simulink model "pi1semanti"  (R2020a)
settings: Solver=VariableStepAuto  StartTime=0.0  StopTime=1  RelTol=1e-3
values from neighbouring files (symbols this model uses):
  B = 0.003032    [motorfase_valores.m]
  flux = 0.12    [motorfase_valores.m]
  inddiff = 0.0125    [motorfase_valores.m]
  J = 0.0042    [motorfase_valores.m]
  p = 3    [motorfase_valores.m]
  R = 2.3    [motorfase_valores.m]
libraries: powerlib x13, eePwmGenerator x1, simulink x1
settings Model: Creator=ryt14  LastModifiedBy=ryt14
settings SolverCC: ZeroCrossAlgorithm=Adaptive
settings DebuggingCC: IgnoredZcDiagnostic=none

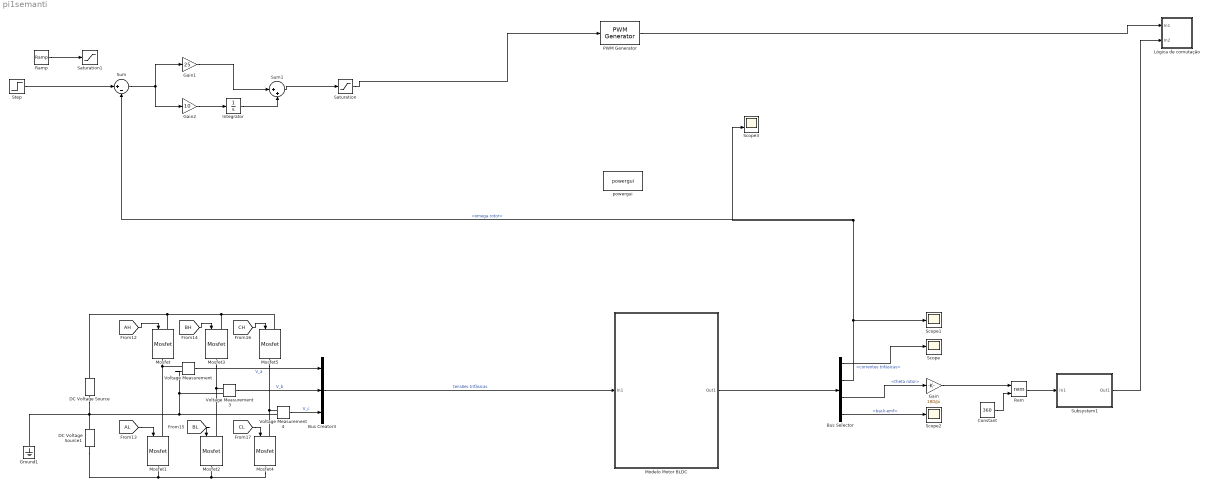
== system pi1semanti ==
  Bus Creator3 : BusCreator  Inputs=3
  Bus Selector : BusSelector  OutputSignals=correntes trifásicas,omega rotor,theta rotor,back-emf
  Constant : Constant  Value=360
  DC Voltage Source : powerlib/Electrical Sources/DC Voltage Source  Amplitude=75  Measurements=None
  DC Voltage Source1 : powerlib/Electrical Sources/DC Voltage Source  Amplitude=75  Measurements=None
  Gain : Gain  Gain=180/pi
  Gain1 : Gain  Gain=25
  Gain2 : Gain  Gain=10
  Ground1 : powerlib/Elements/Ground  LConnTagsString=a
  Integrator : Integrator
  Lógica de comutação : Subsystem
  Modelo Motor BLDC : Subsystem
  Mosfet{,1..5} (6 alike) : powerlib/Power Electronics/Mosfet  Ron=0.1  Lon=0  Rd=0.01  Vfd=0  IC=0  Rs=1e5  Cs=inf  Measurements=off
  PWM Generator : eePwmGenerator/PWM Generator  CarrCount=Up  Tper=0.001  Ts=5e-5
  Ramp : simulink/Sources/Ramp  slope=10  start=0  InitialOutput=0
  Rem : Math  Operator=rem  SaturateOnIntegerOverflow=on
  Saturation : Saturate  UpperLimit=1  LowerLimit=0
  Saturation1 : Saturate  UpperLimit=50  LowerLimit=0
  Scope : Scope
  Scope1 : Scope
  Scope2 : Scope
  Scope3 : Scope  NumInputPorts=2
  Step : Step  Time=0  After=100  SampleTime=0
  Subsystem1 : Subsystem
  Sum : Sum  Inputs=|+-
  Sum1 : Sum  Inputs=|++
  Voltage Measurement : powerlib/Measurements/Voltage Measurement  PhasorSimulation=off  OutputType=Complex  PSBequivalent=0
  Voltage Measurement3 : powerlib/Measurements/Voltage Measurement  PhasorSimulation=off  OutputType=Complex  PSBequivalent=0
  Voltage Measurement4 : powerlib/Measurements/Voltage Measurement  PhasorSimulation=off  OutputType=Complex  PSBequivalent=0
  powergui : powerlib/powergui  Priority=1  SimulationMode=Continuous  SampleTime=50e-6  frequency=60  Iterations=50  frequencyindice=0  Pbase=100e6  ErrMax=1e-4  UnitsV=kV  UnitsW=MW  buscounter=0  FunctionMessages=off  echomessages=off  EnableUseOfTLC=off  CurrentSourceSwitches=off  DisableSnubberDevices=off  DisableRonSwitches=off  DisableVfSwitches=off  DisplayEquations=off  AutomaticDiscreteSolvers=off  SolverType=Tustin/Backward Euler (TBE)  Interpol=off  ExternalGateDelay=off  methode=off  Ts=100  x0status=blocks  SPID=on  SwTol=0  HookPort=off  NonlinearTolerance=1e-4  nMaxIteration=100  ContinueOnMaxIteration=off  RestoreLinks=warning  ResistiveCurrentMeasurement=off  Frange=[0:2:500]  Ylog=off  Xlog=on  ShowGrid=off  save=off  variable=ZData  structure=0  ZoomFFT=off  StartTime=0.0  cycles=1  DisplayStyle=1  fundamental=60  FreqAxis=off  MaxFrequency=1000  frequencyindicesteady=1  RmsSteady=1  display=off
  wires:
  Voltage Measurement3/1 -> Bus Creator3/2  "V_b"
  Voltage Measurement4/1 -> Bus Creator3/3  "V_c"
  Voltage Measurement/1 -> Bus Creator3/1  "V_a"
  Bus Creator3/1 -> Modelo Motor BLDC/1(In1)  "tensões trifásicas"
  Modelo Motor BLDC/1(Out1) -> Bus Selector/1
  Gain/1 -> Rem/1
  Bus Selector/3 -> Gain/1  "<theta rotor>"
  Constant/1 -> Rem/2
  Rem/1 -> Subsystem1/1(In1)
  Bus Selector/2 -> Scope3/2, Sum/2, Scope1/1  "<omega rotor>"
  [AH] -> Mosfet/1
  [BH] -> Mosfet3/1
  [CH] -> Mosfet5/1
  [BL] -> Mosfet2/1
  [CL] -> Mosfet4/1
  [AL] -> Mosfet1/1
  Bus Selector/1 -> Scope/1  "<correntes trifásicas>"
  Bus Selector/4 -> Scope2/1  "<back-emf>"
  Sum/1 -> Gain1/1, Gain2/1
  PWM Generator/1 -> Lógica de comutação/1(In1)
  Subsystem1/1(Out1) -> Lógica de comutação/2(In2)
  Sum1/1 -> Saturation/1
  Saturation/1 -> PWM Generator/1
  Gain1/1 -> Sum1/1
  Integrator/1 -> Sum1/2
  Gain2/1 -> Integrator/1
  Ramp/1 -> Saturation1/1
  Step/1 -> Sum/1
  connections:
  Mosfet/RConn1 -- Mosfet1/LConn1 -- Voltage Measurement/LConn1
  Mosfet3/RConn1 -- Mosfet2/LConn1 -- Voltage Measurement3/LConn1
  Mosfet5/RConn1 -- Mosfet4/LConn1 -- Voltage Measurement4/LConn1
  Mosfet/LConn1 -- Mosfet5/LConn1 -- Mosfet3/LConn1 -- DC Voltage Source/RConn1
  DC Voltage Source/LConn1 -- Ground1/LConn1 -- DC Voltage Source1/RConn1 -- Voltage Measurement3/LConn2 -- Voltage Measurement/LConn2 -- Voltage Measurement4/LConn2
  Mosfet4/RConn1 -- DC Voltage Source1/LConn1 -- Mosfet1/RConn1 -- Mosfet2/RConn1

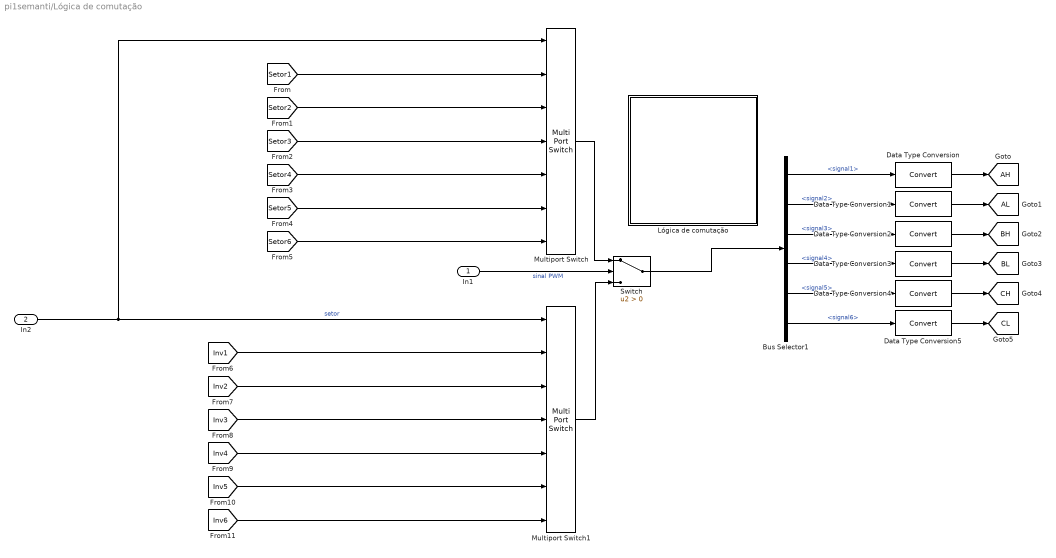
== system pi1semanti/Lógica de comutação ==
  In1 : Inport
  In2 : Inport  Port=2
  Bus Selector1 : BusSelector  OutputSignals=signal1,signal2,signal3,signal4,signal5,signal6
  Data Type Conversion{,1..5} (6 alike) : DataTypeConversion
  Lógica de comutação : Subsystem
  Multiport Switch : MultiPortSwitch  Inputs=6
  Multiport Switch1 : MultiPortSwitch  Inputs=6
  Switch : Switch  Criteria=u2 > Threshold
  tag scope: AH=global, AL=global, BH=global, BL=global, CH=global, CL=global
  wires:
  [Setor5] -> Multiport Switch/6
  [Inv4] -> Multiport Switch1/5
  [Setor1] -> Multiport Switch/2
  Data Type Conversion1/1 -> [AL]
  [Setor3] -> Multiport Switch/4
  Bus Selector1/2 -> Data Type Conversion1/1  "<signal2>"
  Data Type Conversion4/1 -> [CH]
  Switch/1 -> Bus Selector1/1
  [Setor6] -> Multiport Switch/7
  Bus Selector1/5 -> Data Type Conversion4/1  "<signal5>"
  Data Type Conversion/1 -> [AH]
  [Inv3] -> Multiport Switch1/4
  Data Type Conversion5/1 -> [CL]
  Bus Selector1/6 -> Data Type Conversion5/1  "<signal6>"
  Bus Selector1/1 -> Data Type Conversion/1  "<signal1>"
  [Inv2] -> Multiport Switch1/3
  Bus Selector1/3 -> Data Type Conversion2/1  "<signal3>"
  [Setor2] -> Multiport Switch/3
  [Inv1] -> Multiport Switch1/2
  Data Type Conversion3/1 -> [BL]
  Data Type Conversion2/1 -> [BH]
  In2/1 -> Multiport Switch1/1, Multiport Switch/1  "setor"
  Multiport Switch/1 -> Switch/1
  [Setor4] -> Multiport Switch/5
  [Inv6] -> Multiport Switch1/7
  [Inv5] -> Multiport Switch1/6
  Multiport Switch1/1 -> Switch/3
  Bus Selector1/4 -> Data Type Conversion3/1  "<signal4>"
  In1/1 -> Switch/2  "sinal PWM"

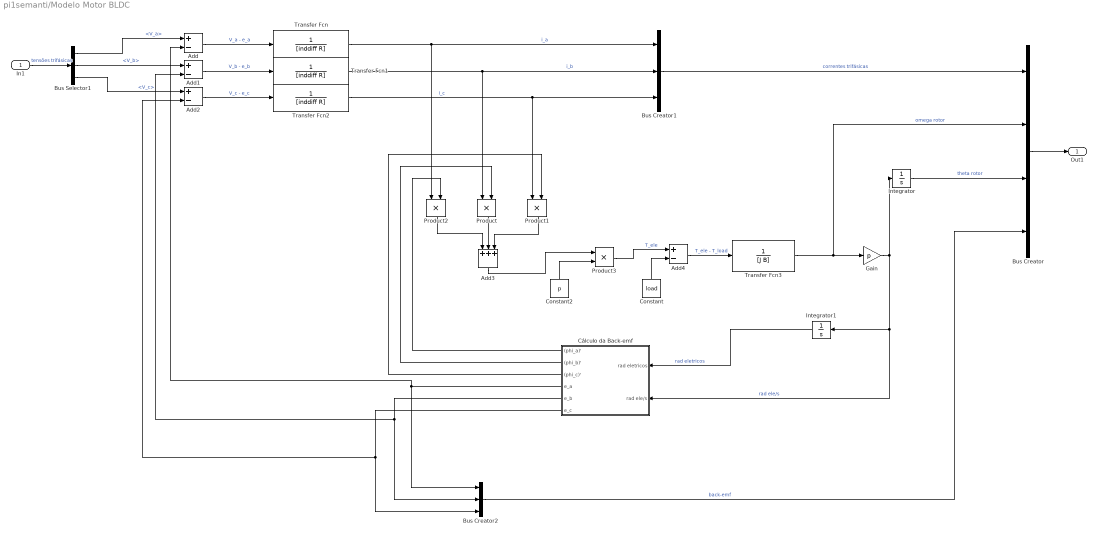
== system pi1semanti/Modelo Motor BLDC ==
  In1 : Inport
  Add{,1..2,4} (4 alike) : Sum  Inputs=+-
  Add3 : Sum  Inputs=+++
  Bus Creator : BusCreator  Inputs=4
  Bus Creator1 : BusCreator  Inputs=3
  Bus Creator2 : BusCreator  Inputs=3
  Bus Selector1 : BusSelector  OutputSignals=V_a,V_b,V_c
  Constant : Constant  Value=load
  Constant2 : Constant  Value=p
  Cálculo da Back-emf : Subsystem
  Gain : Gain  Gain=p
  Integrator : Integrator
  Integrator1 : Integrator
  Product : Product
  Product1 : Product
  Product2 : Product
  Product3 : Product  Inputs=**
  Transfer Fcn : TransferFcn  Denominator=[inddiff R]
  Transfer Fcn1 : TransferFcn  Denominator=[inddiff R]
  Transfer Fcn2 : TransferFcn  Denominator=[inddiff R]
  Transfer Fcn3 : TransferFcn  Denominator=[J B]
  Out1 : Outport
  wires:
  Add/1 -> Transfer Fcn/1  "V_a - e_a"
  Add2/1 -> Transfer Fcn2/1  "V_c - e_c"
  Constant/1 -> Add4/2
  Bus Selector1/2 -> Add1/1  "<V_b>"
  Bus Creator1/1 -> Bus Creator/1  "correntes trifásicas"
  Add1/1 -> Transfer Fcn1/1  "V_b - e_b"
  Product1/1 -> Add3/3
  Transfer Fcn1/1 -> Product/1, Bus Creator1/2  "i_b"
  Product2/1 -> Add3/1
  Product3/1 -> Add4/1  "T_ele"
  Bus Selector1/1 -> Add/1  "<V_a>"
  Transfer Fcn2/1 -> Product1/1, Bus Creator1/3  "i_c"
  Add4/1 -> Transfer Fcn3/1  "T_ele - T_load"
  Transfer Fcn/1 -> Product2/1, Bus Creator1/1  "i_a"
  Bus Selector1/3 -> Add2/1  "<V_c>"
  Bus Creator2/1 -> Bus Creator/4  "back-emf"
  Product/1 -> Add3/2
  In1/1 -> Bus Selector1/1  "tensões trifásicas"
  Gain/1 -> Integrator/1, Integrator1/1, Cálculo da Back-emf/2(rad ele/s)  "rad ele/s"
  Integrator/1 -> Bus Creator/3  "theta rotor"
  Bus Creator/1 -> Out1/1
  Add3/1 -> Product3/1
  Constant2/1 -> Product3/2
  Transfer Fcn3/1 -> Bus Creator/2, Gain/1  "omega rotor"
  Cálculo da Back-emf/6(e_c) -> Add2/2, Bus Creator2/3
  Cálculo da Back-emf/5(e_b) -> Add1/2, Bus Creator2/2
  Cálculo da Back-emf/4(e_a) -> Add/2, Bus Creator2/1
  Integrator1/1 -> Cálculo da Back-emf/1(rad eletricos)  "rad eletricos"
  Cálculo da Back-emf/1((phi_a)') -> Product2/2
  Cálculo da Back-emf/2((phi_b)') -> Product/2
  Cálculo da Back-emf/3((phi_c)') -> Product1/2

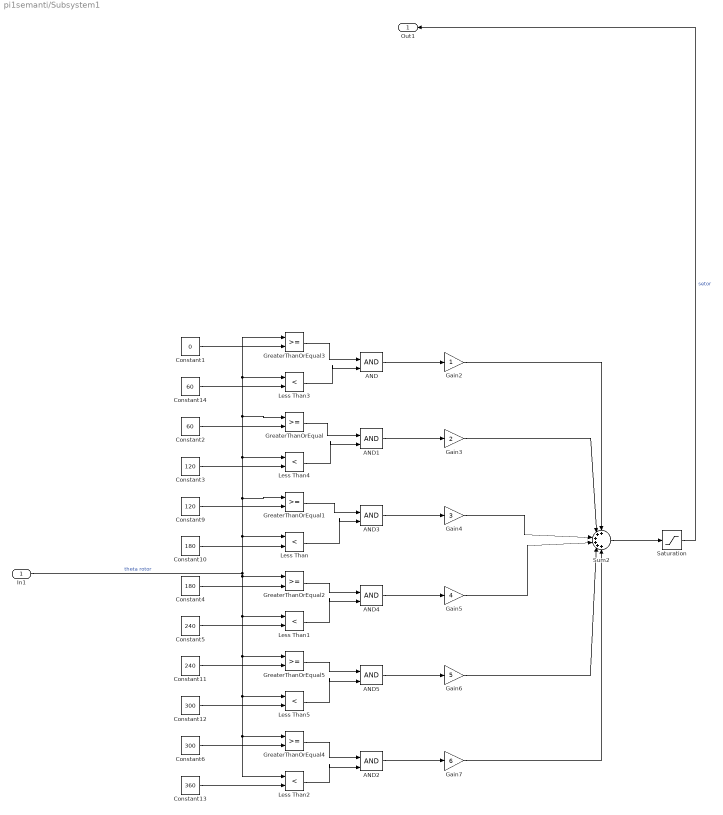
== system pi1semanti/Subsystem1 ==
  In1 : Inport
  AND{,1..5} (6 alike) : Logic  IconShape=distinctive  AllPortsSameDT=off  OutDataTypeStr=boolean
  Constant1 : Constant  Value=0
  Constant10 : Constant  Value=180
  Constant11 : Constant  Value=240
  Constant12 : Constant  Value=300
  Constant13 : Constant  Value=360
  Constant14 : Constant  Value=60
  Constant2 : Constant  Value=60
  Constant3 : Constant  Value=120
  Constant4 : Constant  Value=180
  Constant5 : Constant  Value=240
  Constant6 : Constant  Value=300
  Constant9 : Constant  Value=120
  Gain2 : Gain
  Gain3 : Gain  Gain=2
  Gain4 : Gain  Gain=3
  Gain5 : Gain  Gain=4
  Gain6 : Gain  Gain=5
  Gain7 : Gain  Gain=6
  GreaterThanOrEqual{,1..5} (6 alike) : RelationalOperator  OutDataTypeStr=boolean  RndMeth=Simplest
  Less Than{,1..5} (6 alike) : RelationalOperator  Operator=<  OutDataTypeStr=boolean  RndMeth=Simplest
  Saturation : Saturate  UpperLimit=6  LowerLimit=1
  Sum2 : Sum  Inputs=++++++
  Out1 : Outport
  wires:
  In1/1 -> Less Than/1, GreaterThanOrEqual1/1, GreaterThanOrEqual/1, GreaterThanOrEqual3/1, Less Than3/1, Less Than4/1, Less Than2/1, GreaterThanOrEqual4/1, Less Than5/1, GreaterThanOrEqual5/1, Less Than1/1, GreaterThanOrEqual2/1  "theta rotor"
  Less Than1/1 -> AND4/2
  Gain2/1 -> Sum2/1
  Sum2/1 -> Saturation/1
  Constant1/1 -> GreaterThanOrEqual3/2
  Constant9/1 -> GreaterThanOrEqual1/2
  Gain4/1 -> Sum2/3
  Gain5/1 -> Sum2/4
  AND/1 -> Gain2/1
  Constant13/1 -> Less Than2/2
  Constant2/1 -> GreaterThanOrEqual/2
  AND4/1 -> Gain5/1
  AND1/1 -> Gain3/1
  Less Than5/1 -> AND5/2
  Less Than/1 -> AND3/2
  GreaterThanOrEqual1/1 -> AND3/1
  Constant4/1 -> GreaterThanOrEqual2/2
  Gain3/1 -> Sum2/2
  Less Than2/1 -> AND2/2
  GreaterThanOrEqual5/1 -> AND5/1
  GreaterThanOrEqual/1 -> AND1/1
  Gain6/1 -> Sum2/5
  AND2/1 -> Gain7/1
  AND5/1 -> Gain6/1
  Less Than3/1 -> AND/2
  Constant11/1 -> GreaterThanOrEqual5/2
  Constant12/1 -> Less Than5/2
  Constant3/1 -> Less Than4/2
  Constant5/1 -> Less Than1/2
  Saturation/1 -> Out1/1  "setor"
  AND3/1 -> Gain4/1
  Constant14/1 -> Less Than3/2
  GreaterThanOrEqual2/1 -> AND4/1
  Less Than4/1 -> AND1/2
  Constant6/1 -> GreaterThanOrEqual4/2
  Constant10/1 -> Less Than/2
  GreaterThanOrEqual4/1 -> AND2/1
  Gain7/1 -> Sum2/6
  GreaterThanOrEqual3/1 -> AND/1

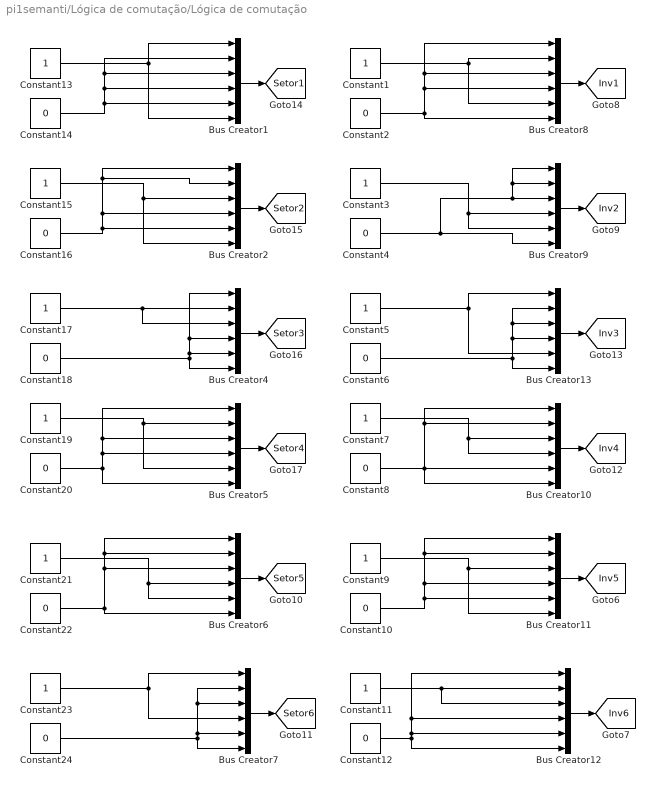
== system pi1semanti/Lógica de comutação/Lógica de comutação ==
  Bus Creator{1..2,4..13} (12 alike) : BusCreator  Inputs=6
  Constant{1,3,5,7,9,11,13,15,17,19,21,23} (12 alike) : Constant
  Constant{2,4,6,8,10,12,14,16,18,20,22,24} (12 alike) : Constant  Value=0
  tag scope: Inv1=global, Inv2=global, Inv3=global, Inv4=global, Inv5=global, Inv6=global, Setor1=global, Setor2=global, Setor3=global, Setor4=global, Setor5=global, Setor6=global
  wires:
  Bus Creator12/1 -> [Inv6]
  Constant24/1 -> Bus Creator7/6, Bus Creator7/5, Bus Creator7/3, Bus Creator7/2
  Bus Creator9/1 -> [Inv2]
  Constant16/1 -> Bus Creator2/4, Bus Creator2/2, Bus Creator2/1, Bus Creator2/5
  Constant6/1 -> Bus Creator13/6, Bus Creator13/3, Bus Creator13/2, Bus Creator13/4
  Constant1/1 -> Bus Creator8/2, Bus Creator8/5
  Constant4/1 -> Bus Creator9/1, Bus Creator9/2, Bus Creator9/3, Bus Creator9/6
  Bus Creator7/1 -> [Setor6]
  Constant18/1 -> Bus Creator4/6, Bus Creator4/5, Bus Creator4/4, Bus Creator4/1
  Constant12/1 -> Bus Creator12/5, Bus Creator12/1, Bus Creator12/4, Bus Creator12/6
  Constant23/1 -> Bus Creator7/4, Bus Creator7/1
  Constant7/1 -> Bus Creator10/4, Bus Creator10/3
  Constant10/1 -> Bus Creator11/1, Bus Creator11/2, Bus Creator11/4, Bus Creator11/5
  Constant3/1 -> Bus Creator9/5, Bus Creator9/4
  Constant15/1 -> Bus Creator2/6, Bus Creator2/3
  Bus Creator5/1 -> [Setor4]
  Constant8/1 -> Bus Creator10/2, Bus Creator10/1, Bus Creator10/5, Bus Creator10/6
  Constant2/1 -> Bus Creator8/6, Bus Creator8/3, Bus Creator8/1, Bus Creator8/4
  Bus Creator6/1 -> [Setor5]
  Constant17/1 -> Bus Creator4/3, Bus Creator4/2
  Bus Creator4/1 -> [Setor3]
  Constant19/1 -> Bus Creator5/2, Bus Creator5/5
  Constant5/1 -> Bus Creator13/1, Bus Creator13/5
  Bus Creator11/1 -> [Inv5]
  Bus Creator1/1 -> [Setor1]
  Bus Creator8/1 -> [Inv1]
  Bus Creator2/1 -> [Setor2]
  Bus Creator10/1 -> [Inv4]
  Constant21/1 -> Bus Creator6/5, Bus Creator6/4
  Bus Creator13/1 -> [Inv3]
  Constant22/1 -> Bus Creator6/6, Bus Creator6/3, Bus Creator6/2, Bus Creator6/1
  Constant20/1 -> Bus Creator5/6, Bus Creator5/4, Bus Creator5/1, Bus Creator5/3
  Constant9/1 -> Bus Creator11/6, Bus Creator11/3
  Constant11/1 -> Bus Creator12/3, Bus Creator12/2
  Constant13/1 -> Bus Creator1/1, Bus Creator1/6
  Constant14/1 -> Bus Creator1/4, Bus Creator1/2, Bus Creator1/3, Bus Creator1/5

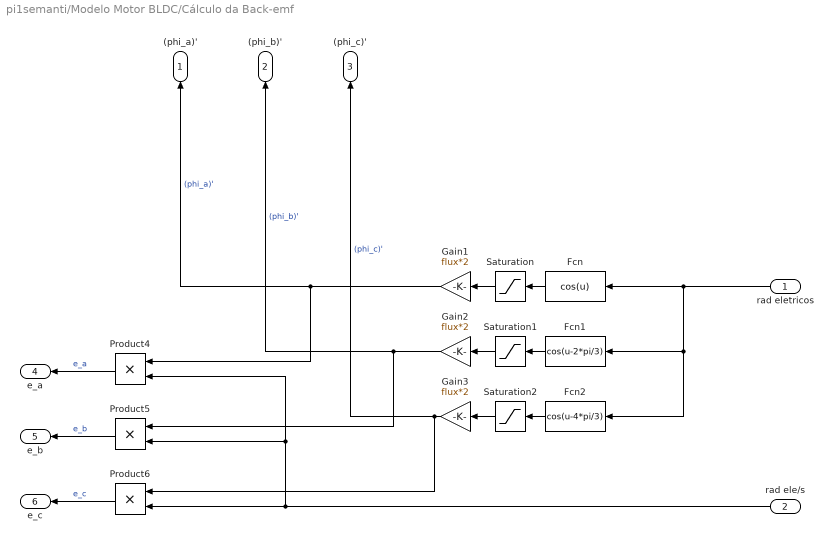
== system pi1semanti/Modelo Motor BLDC/Cálculo da Back-emf ==
  rad eletricos : Inport
  rad ele/s : Inport  Port=2
  Fcn : Fcn  Expr=cos(u)
  Fcn1 : Fcn  Expr=cos(u-2*pi/3)
  Fcn2 : Fcn  Expr=cos(u-4*pi/3)
  Gain1 : Gain  Gain=flux*2
  Gain2 : Gain  Gain=flux*2
  Gain3 : Gain  Gain=flux*2
  Product4 : Product
  Product5 : Product
  Product6 : Product
  Saturation : Saturate
  Saturation1 : Saturate
  Saturation2 : Saturate
  (phi_a)' : Outport
  (phi_b)' : Outport  Port=2
  (phi_c)' : Outport  Port=3
  e_a : Outport  Port=4
  e_b : Outport  Port=5
  e_c : Outport  Port=6
  wires:
  Saturation/1 -> Gain1/1
  rad ele/s/1 -> Product5/2, Product4/2, Product6/2
  Product4/1 -> e_a/1  "e_a"
  Fcn1/1 -> Saturation1/1
  Gain2/1 -> (phi_b)'/1, Product5/1  "(phi_b)'"
  Fcn/1 -> Saturation/1
  Fcn2/1 -> Saturation2/1
  Gain1/1 -> (phi_a)'/1, Product4/1  "(phi_a)'"
  Gain3/1 -> (phi_c)'/1, Product6/1  "(phi_c)'"
  rad eletricos/1 -> Fcn2/1, Fcn1/1, Fcn/1
  Saturation1/1 -> Gain2/1
  Saturation2/1 -> Gain3/1
  Product5/1 -> e_b/1  "e_b"
  Product6/1 -> e_c/1  "e_c"
